simulink subsystem "InjectorOmega"  (R2020b)
settings: Solver=VariableStepAuto  StartTime=0.0  StopTime=10.0  RelTol=1e-3
model mask{CdOmegaLow=0.85, CdOmegaHigh=0.73, KExcessPressureDrop=2.28, numHolesPort1=5, numHolesPort2=5, holeDiamPort1=1.5e-3, holeDiamPort2=1.5e-3, LInjector=5e-3}
  mask prompts: CdOmegaLow "Cd used for omega with low supercharge. UofT recommends 0.85"; CdOmegaHigh "Cd used for omega with high supercharge. UofT recommends 0.73"; KExcessPressureDrop "K Excess pressure drop constant used with Dyer for Cd calculation. Langhaar says 2.28 for sharp edge inlets"; numHolesPort1 "Number of holes port 1"; numHolesPort2 "Number of holes port 2"; holeDiamPort1 "Single hole diameter port 1 (m)"; holeDiamPort2 "Single hole diameter port 2 (m)"; LInjector "L Injector Depth (m)"
libraries: nesl_utility x3, fl_lib x3, SimscapeCustomBlocks_lib x2
settings Model: Creator=Edward  LastModifiedBy=Edward

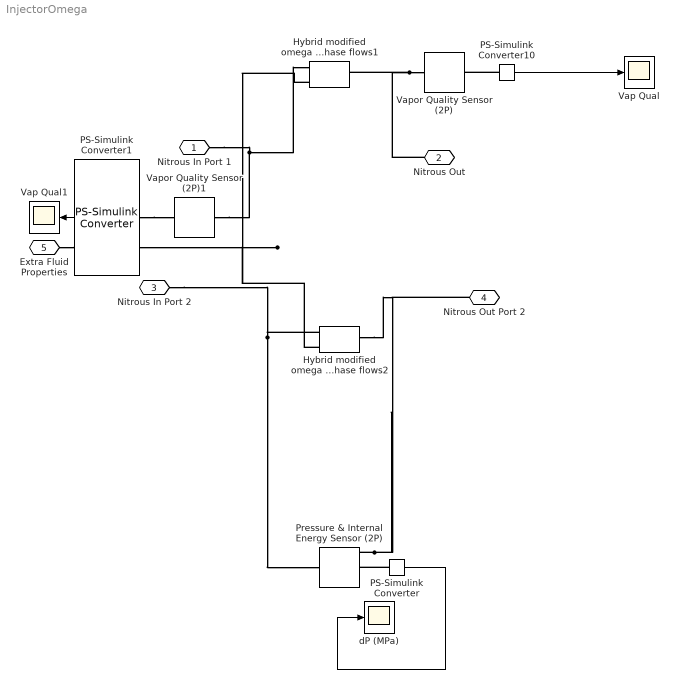
== system InjectorOmega ==
  Hybrid modified omega and NHNE (Dyer) Orifice for cavitating and/or super charged liquid or two phase flows1 : SimscapeCustomBlocks_lib/Hybrid modified omega and NHNE (Dyer) Orifice for cavitating and//or super charged liquid or two phase flows  area=Sim.preInjectorPipe.crossSection m^2  orifice_area=numHolesPort1 * 0.25*pi*(holeDiamPort1)^2 m^2  injector_depth=LInjector m  single_hole_diam=holeDiamPort1 m  K_excess=KExcessPressureDrop  CdOmegaLow=CdOmegaLow  CdOmegaHigh=CdOmegaHigh
      settings: InternalSimscapePortConfiguration="{\"Bottom\":[],\"Left\":[{\"id\":\"A\",\"label\":\"A\",\"type\":\"foundation.two_phase_fluid.two_phase_fluid\"}],\"Right\":[{\"id\":\"B\",\"label\":\"B\",\"type\":\"foundation.two_phase_fluid.two_phase_fluid\"}],\"Top\":[{\"id\":\"Props\",\"label\":\"Props\",\"type\":\"SimscapeCustomBlocks.customFluidDomain.extra_two_phase_fluid_props\"}]}"
  Hybrid modified omega and NHNE (Dyer) Orifice for cavitating and/or super charged liquid or two phase flows2 : SimscapeCustomBlocks_lib/Hybrid modified omega and NHNE (Dyer) Orifice for cavitating and//or super charged liquid or two phase flows  area=Sim.preInjectorPipe.crossSection m^2  orifice_area=numHolesPort2 * 0.25*pi*(holeDiamPort2)^2 m^2  injector_depth=LInjector m  single_hole_diam=holeDiamPort2 m  K_excess=KExcessPressureDrop  CdOmegaLow=CdOmegaLow  CdOmegaHigh=CdOmegaHigh
      settings: InternalSimscapePortConfiguration="{\"Bottom\":[],\"Left\":[{\"id\":\"A\",\"label\":\"A\",\"type\":\"foundation.two_phase_fluid.two_phase_fluid\"}],\"Right\":[{\"id\":\"B\",\"label\":\"B\",\"type\":\"foundation.two_phase_fluid.two_phase_fluid\"}],\"Top\":[{\"id\":\"Props\",\"label\":\"Props\",\"type\":\"SimscapeCustomBlocks.customFluidDomain.extra_two_phase_fluid_props\"}]}"
  PS-Simulink Converter : nesl_utility/PS-Simulink Converter  PhysicalDomain=network_engine_domain  SubClassName=ps_output  LeftPortType=input  RightPortType=output  PseudoPeriodic=off  Frequencies=[]  Unit=inherit  AffineConversion=off
  PS-Simulink Converter1 : nesl_utility/PS-Simulink Converter  PhysicalDomain=network_engine_domain  SubClassName=ps_output  LeftPortType=input  RightPortType=output  PseudoPeriodic=off  Frequencies=[]  Unit=inherit  AffineConversion=off
  PS-Simulink Converter10 : nesl_utility/PS-Simulink Converter  PhysicalDomain=network_engine_domain  SubClassName=ps_output  LeftPortType=input  RightPortType=output  PseudoPeriodic=off  Frequencies=[]  Unit=inherit  AffineConversion=off
  Pressure & Internal Energy Sensor (2P) : fl_lib/Two-Phase Fluid/Sensors/Pressure & Internal Energy Sensor (2P)
      settings: SourceProductBaseCode=SS  InternalSimscapePortConfiguration="{\"Bottom\":[],\"Left\":[{\"id\":\"A\",\"label\":\"A\",\"type\":\"foundation.two_phase_fluid.two_phase_fluid\"}],\"Right\":[{\"id\":\"B\",\"label\":\"B\",\"type\":\"foundation.two_phase_fluid.two_phase_fluid\"},{\"id\":\"P\",\"label\":\"P\",\"type\":\"output\"},{\"id\":\"U\",\"label\":\"U\",\"type\":\"output\"}],\"Top\":[]}"
  Vap Qual : Scope
  Vap Qual1 : Scope
  Vapor Quality Sensor (2P) : fl_lib/Two-Phase Fluid/Sensors/Vapor Quality Sensor (2P)  vapor_fraction_spec=foundation.enum.vapor_fraction_spec.quality
      settings: SourceProductBaseCode=SS  InternalSimscapePortConfiguration="{\"Bottom\":[],\"Left\":[{\"id\":\"A\",\"label\":\"A\",\"type\":\"foundation.two_phase_fluid.two_phase_fluid\"}],\"Right\":[{\"id\":\"X\",\"label\":\"X\",\"type\":\"output\"}],\"Top\":[]}"
  Vapor Quality Sensor (2P)1 : fl_lib/Two-Phase Fluid/Sensors/Vapor Quality Sensor (2P)  vapor_fraction_spec=foundation.enum.vapor_fraction_spec.quality
      settings: SourceProductBaseCode=SS  InternalSimscapePortConfiguration="{\"Bottom\":[],\"Left\":[{\"id\":\"A\",\"label\":\"A\",\"type\":\"foundation.two_phase_fluid.two_phase_fluid\"}],\"Right\":[{\"id\":\"X\",\"label\":\"X\",\"type\":\"output\"}],\"Top\":[]}"
  dP (MPa) : Scope
  Nitrous In Port 1 : PMIOPort  Side=Left
  Nitrous Out : PMIOPort  Port=2  Side=Right
  Nitrous In Port 2 : PMIOPort  Port=3  Side=Left
  Nitrous Out Port 2 : PMIOPort  Port=4  Side=Right
  Extra Fluid Properties : PMIOPort  Port=5  Side=Left
  wires:
  PS-Simulink Converter1/1 -> Vap Qual1/1
  PS-Simulink Converter10/1 -> Vap Qual/1
  PS-Simulink Converter/1 -> dP (MPa)/1
  connections:
  Pressure & Internal Energy Sensor (2P)/RConn1 -- Hybrid modified omega and NHNE (Dyer) Orifice for cavitating and/or super charged liquid or two phase flows2/RConn1 -- Nitrous Out Port 2/RConn1
  Nitrous In Port 2/RConn1 -- Hybrid modified omega and NHNE (Dyer) Orifice for cavitating and/or super charged liquid or two phase flows2/LConn1 -- Pressure & Internal Energy Sensor (2P)/LConn1
  Nitrous In Port 1/RConn1 -- Hybrid modified omega and NHNE (Dyer) Orifice for cavitating and/or super charged liquid or two phase flows1/LConn1 -- Vapor Quality Sensor (2P)1/LConn1
  Vapor Quality Sensor (2P)/LConn1 -- Hybrid modified omega and NHNE (Dyer) Orifice for cavitating and/or super charged liquid or two phase flows1/RConn1 -- Nitrous Out/RConn1
  Extra Fluid Properties/RConn1 -- Hybrid modified omega and NHNE (Dyer) Orifice for cavitating and/or super charged liquid or two phase flows2/LConn2 -- Hybrid modified omega and NHNE (Dyer) Orifice for cavitating and/or super charged liquid or two phase flows1/LConn2
  PS-Simulink Converter1/LConn1 -- Vapor Quality Sensor (2P)1/RConn1
  PS-Simulink Converter10/LConn1 -- Vapor Quality Sensor (2P)/RConn1
  PS-Simulink Converter/LConn1 -- Pressure & Internal Energy Sensor (2P)/RConn2
